simulink model "p2simulink"  (Simulink 9.1)
settings: Solver=VariableStepAuto  StartTime=0.0  StopTime=10.0  RelTol=1e-3
values from neighbouring files (symbols this model uses):
  b = 0.5    [Problema2.m]    (also in Problema2TF.m)
  e = eps    [Problema2.m]    (also in Problema2TF.m)
  g = 9.8    [Problema2.m]    (also in Problema2TF.m)
  k = 2    [Problema2.m]    (also in Problema2TF.m)
  L = 0.01    [Problema2.m]    (also in Problema2TF.m)
  m = 0.2    [Problema2.m]    (also in Problema2TF.m; criterioRouth.m = 4)
  R = 20    [Problema2.m]    (also in Problema2TF.m)
undefined symbols (not defined in the file or in its folder): magnitude
settings Model: Creator=valen  LastModifiedBy=valen
settings DataIOCC: SaveFormat=Dataset
settings OptimizationCC: LifeSpan=auto
settings DebuggingCC: UnderspecifiedInitializationDetection=Simplified  MergeDetectMultiDrivingBlocksExec=error  SFUnexpectedBacktrackingDiag=error  SFNoUnconditionalDefaultTransitionDiag=error  SFExecutionAtInitializationDiag=warning
settings HardwareCC: ProdBitPerPointer=64  ProdBitPerSizeT=64  ProdBitPerPtrDiffT=64  ProdLargestAtomicFloat=Float  ProdIntDivRoundTo=Zero  ProdEndianess=LittleEndian  ProdWordSize=64  ProdHWDeviceType=Intel->x86-64 (Windows64)
settings ModelReferenceCC: PropagateSignalLabelsOutOfModel=on
settings CodeAppCC: StateflowObjectComments=off
settings GRTTargetCC: TargetLangStandard=C99 (ISO)  CombineOutputUpdateFcns=on  GRTInterface=off
settings ConfigComp: CovMetricSettings=dwe  CovHtmlReporting=off  CovSaveCumulativeToWorkspaceVar=off  CovSaveSingleToWorkspaceVar=off  CovExternalEMLEnable=on

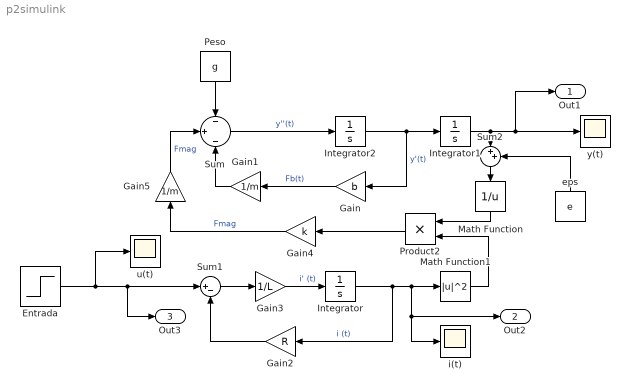
== system p2simulink ==
  Entrada : Step  Time=100  Before=12  After=12  SampleTime=0
  Gain : Gain  Gain=b
  Gain1 : Gain  Gain=1/m
  Gain2 : Gain  Gain=R
  Gain3 : Gain  Gain=1/L
  Gain4 : Gain  Gain=k
  Gain5 : Gain  Gain=1/m
  Integrator : Integrator  InitialCondition=0.5
  Integrator1 : Integrator  InitialCondition=0.2551
  Integrator2 : Integrator
  Math Function : Math  Operator=reciprocal  SaturateOnIntegerOverflow=on
  Math Function1 : Math  Operator=magnitude^2  SaturateOnIntegerOverflow=on
  Peso : Constant  Value=g
  Product2 : Product
  Sum : Sum  Inputs=-|+|-
  Sum1 : Sum  Inputs=|+-
  Sum2 : Sum  Inputs=|++
  eps : Constant  Value=e
  i(t) : Scope
  u(t) : Scope
  y(t) : Scope
  Out1 : Outport
  Out2 : Outport  Port=2
  Out3 : Outport  Port=3
  wires:
  Integrator2/1 -> Integrator1/1, Gain/1  "y'(t)"
  Sum/1 -> Integrator2/1  "y''(t)"
  Peso/1 -> Sum/1
  Gain3/1 -> Integrator/1  "i' (t)"
  Gain2/1 -> Sum1/2
  Sum1/1 -> Gain3/1
  Entrada/1 -> u(t)/1, Out3/1, Sum1/1
  Integrator1/1 -> Sum2/1, Out1/1, y(t)/1
  Math Function/1 -> Product2/1
  Product2/1 -> Gain4/1
  Math Function1/1 -> Product2/2
  Sum2/1 -> Math Function/1
  eps/1 -> Sum2/2
  Integrator/1 -> Out2/1, i(t)/1, Math Function1/1, Gain2/1  "i (t)"
  Gain4/1 -> Gain5/1  "Fmag"
  Gain5/1 -> Sum/2  "Fmag"
  Gain/1 -> Gain1/1  "Fb(t)"
  Gain1/1 -> Sum/3
